simulink model "Pv"  (R2015a)
settings: Solver=ode45  StartTime=0.0  StopTime=3  RelTol=1e-3
values from neighbouring files (symbols this model uses):
  Iph_array = Iph*Npar    (= 29.801)    [sunpower305.m]
  Isat_array = Isat*Npar    (= 5.8765e-08)    [sunpower305.m]
  Rp_array = Rp*Nser/Npar    (= 198.702)    [sunpower305.m]
  Rs_array = Rs*Nser/Npar    (= 0.0075996)    [sunpower305.m]
  Ts = Ts_Power    (= 1e-06)    [sunpower305.m]
  Ts_Control = 100e-6    (= 0.0001)    [sunpower305.m]
  Ts_Power = 1e-6    (= 1e-06)    [sunpower305.m]
  VT_array = VT*Nser    (= 3.20466023218)    [sunpower305.m]
undefined symbols (not defined in the file or in its folder): sigbuilder_block
libraries: powerlib x16, simulink x2, powerlib_extras x1
settings Model: SimulationMode=accelerator  Creator=Limon  LastModifiedBy=Limon

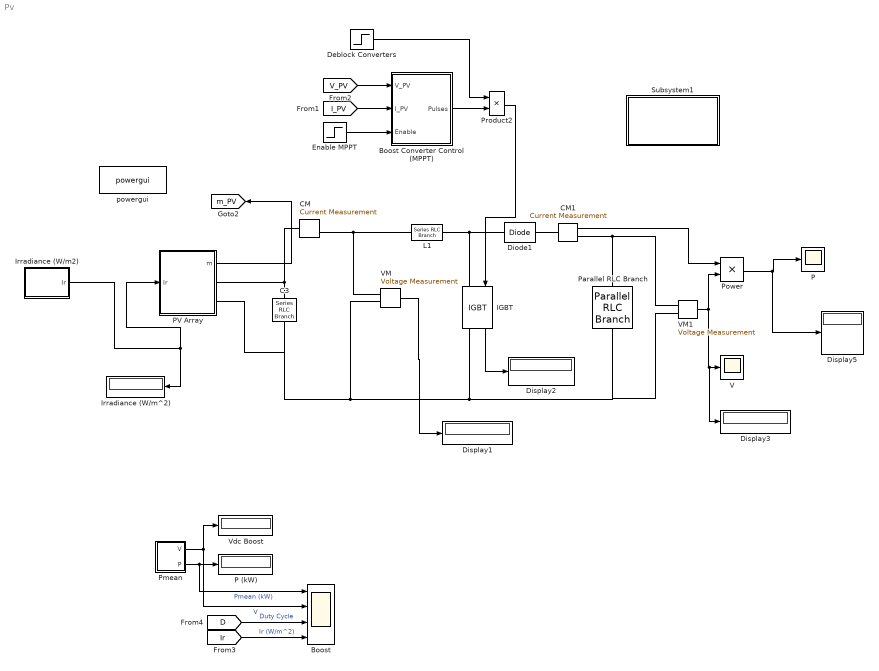
== system Pv ==
  Boost : Scope  NumInputPorts=4
      settings: TimeRange=3  YMin=0~-50~0~200  YMax=35~200~1~1000  SaveName=ScopeData_Boost  Decimation=100  SampleInput=on  SampleTime=Ts_Control
  Boost Converter Control (MPPT) : Subsystem
  C3 : powerlib/Elements/Series RLC Branch  LConnTagsString=__new0  RConnTagsString=__new0  BranchType=C  Resistance=1.0  Inductance=1.0  SetiL0=off  InitialCurrent=0  Capacitance=100e-6  Setx0=off  InitialVoltage=0  Measurements=Branch voltage
  CM : powerlib/Measurements/Current Measurement  PhasorSimulation=off  OutputType=Complex  PSBequivalent=0
  CM1 : powerlib/Measurements/Current Measurement  PhasorSimulation=off  OutputType=Complex  PSBequivalent=0
  Deblock Converters : Step  Time=0.05  SampleTime=0
  Diode1 : powerlib/Power Electronics/Diode  Ron=1e-4  Lon=0  Vf=0  IC=0  UseSnubber=off  Rs=inf  Cs=inf  Measurements=off
  Display{1..3,5} (4 alike) : Display
  Enable MPPT : Step  Time=0.4  SampleTime=0
  IGBT : powerlib/Power Electronics/IGBT  Ron=0.001  Lon=0  Vf=0  Tf=0  Tt=0  IC=0  Rs=1e5  Cs=inf  Measurements=on
  "Irradiance (W/m2) " : Subsystem  Tag=STV Subsys  LoadFcn=sigbuilder_block('load');  StartFcn=sigbuilder_block('start');  StopFcn=sigbuilder_block('stop');  ClipboardFcn=sigbuilder_block('clipboard');  mask(Sigbuilder block){}
      mask help: Sigbuilder GUI
      mask init:
      | if ~strcmp(get_param(bdroot(gcbh),'SimulationStatus'),'stopped') tuvar = sigbuilder_block('maskInit'); end
      settings: CopyFcn=sigbuilder_block('copy');  DeleteFcn=sigbuilder_block('delete');  ModelCloseFcn=sigbuilder_block('modelClose');  PreSaveFcn=sigbuilder_block('preSave');  PauseFcn=sigbuilder_block('pause')  ContinueFcn=sigbuilder_block('continue')  NameChangeFcn=sigbuilder_block('namechange');  OpenFcn=sigbuilder_block('open',[9 136.5 954 513.75 ]);  CloseFcn=sigbuilder_block('close');
      mask Display: plot(0,0,100,100,[10,10,40,40,10],[80,20,20,80,80],[40,10],[50,50], [40,27,10],[65,72,56],[40,25,25,10],[28,28,43,43]);
  Irradiance (W/m^2) : Display
      settings: Format=bank  Decimation=1000
  L1 : powerlib/Elements/Series RLC Branch  LConnTagsString=__new0  RConnTagsString=__new0  BranchType=RL  Resistance=0.005  Inductance=5e-3  SetiL0=off  InitialCurrent=0  Capacitance=1e-6  Setx0=off  InitialVoltage=0  Measurements=None
  P : Scope
      settings: TimeRange=1  YMin=-0  YMax=6e+06  SaveName=ScopeData4
  "P (kW) " : Display
      settings: Format=bank  Decimation=2000
  PV Array : Subsystem
  Parallel RLC Branch : powerlib/Elements/Parallel RLC Branch  LConnTagsString=a  RConnTagsString=__new0  BranchType=RC  Resistance=1e3  Inductance=1e-3  SetiL0=off  InitialCurrent=0  Capacitance=1e-6  Setx0=off  InitialVoltage=0  Measurements=None
  Pmean : Subsystem
  Power : Product
  Product2 : Product  RndMeth=Zero
  Subsystem1 : Subsystem
      mask Display: disp('Measurements')
  V : Scope
      settings: TimeRange=1  YMin=0  YMax=2100  SaveName=ScopeData2
  VM : powerlib/Measurements/Voltage Measurement  PhasorSimulation=off  OutputType=Complex  PSBequivalent=0
  VM1 : powerlib/Measurements/Voltage Measurement  PhasorSimulation=off  OutputType=Complex  PSBequivalent=0
  Vdc Boost : Display
      settings: Format=bank  Decimation=2000
  powergui : powerlib/powergui  Priority=1  SimulationMode=Discrete  SolverType=Tustin  SampleTime=Ts_Power  frequency=60  SPID=off  DisableSnubberDevices=off  DisableRonSwitches=off  DisableVfSwitches=off  SwTol=0  DisplayEquations=off  Interpol=off  methode=off  Ts=0  FunctionMessages=off  echomessages=off  HookPort=off  EnableUseOfTLC=off  x0status=blocks  frequencyindice=0  Pbase=100e6  ErrMax=1e-4  Iterations=50  UnitsV=kV  UnitsW=MW  buscounter=0  RestoreLinks=warning  ResistiveCurrentMeasurement=off  Frange=[0:2:500]  Ylog=off  Xlog=on  ShowGrid=off  save=off  variable=ZData  structure=0  ZoomFFT=on  StartTime=0.0  cycles=1  DisplayStyle=1  fundamental=60  FreqAxis=off  MaxFrequency=1000  frequencyindicesteady=1  RmsSteady=1  display=off
  tag scope: m_PV=global
  wires:
  IGBT/1 -> Display2/1
  VM1/1 -> Power/2, Display3/1, V/1
  CM1/1 -> Power/1
  Power/1 -> Display5/1, P/1
  VM/1 -> Display1/1
  "Irradiance (W/m2) "/1(Ir) -> Irradiance (W/m^2)/1, PV Array/1(Ir)
  PV Array/1(m) -> [m_PV]
  Pmean/2(P) -> "P (kW) "/1, Boost/1  "Pmean (kW)"
  Pmean/1(V) -> Vdc Boost/1, Boost/2  "V"
  [D] -> Boost/3  "Duty Cycle"
  [Ir] -> Boost/4  "Ir (W/m^2)"
  Product2/1 -> IGBT/1
  Deblock Converters/1 -> Product2/1
  Boost Converter Control (MPPT)/1(Pulses) -> Product2/2
  [V_PV] -> Boost Converter Control (MPPT)/1(V_PV)
  [I_PV] -> Boost Converter Control (MPPT)/2(I_PV)
  Enable MPPT/1 -> Boost Converter Control (MPPT)/3(Enable)
  connections:
  C3/LConn1 -- CM/LConn1 -- PV Array/RConn1
  VM/LConn2 -- PV Array/RConn2 -- C3/RConn1 -- VM1/LConn2 -- Parallel RLC Branch/RConn1 -- IGBT/RConn1
  IGBT/LConn1 -- L1/RConn1 -- Diode1/LConn1
  VM/LConn1 -- L1/LConn1 -- CM/RConn1
  CM1/LConn1 -- Diode1/RConn1
  Parallel RLC Branch/LConn1 -- VM1/LConn1 -- CM1/RConn1

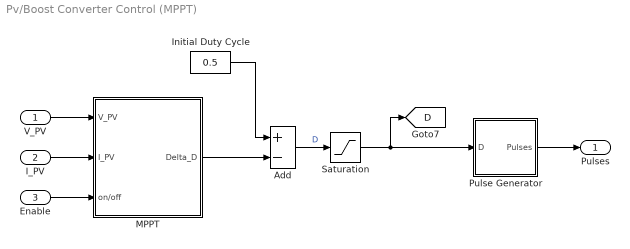
== system Pv/Boost Converter Control (MPPT) ==
  V_PV : Inport
  I_PV : Inport  Port=2
  Enable : Inport  Port=3
  Add : Sum  Inputs=+-
  Initial Duty Cycle : Constant  Value=0.5
  MPPT : Subsystem
  Pulse Generator : Subsystem  mask{Freq=5000}
      mask prompts: Freq "Frequency (Hz)"
  Saturation : Saturate  UpperLimit=1  LowerLimit=0
  Pulses : Outport
  tag scope: D=global
  wires:
  Initial Duty Cycle/1 -> Add/1
  MPPT/1(Delta_D) -> Add/2
  Add/1 -> Saturation/1  "D"
  Saturation/1 -> Pulse Generator/1(D), [D]
  Enable/1 -> MPPT/3(on/off)
  Pulse Generator/1(Pulses) -> Pulses/1
  I_PV/1 -> MPPT/2(I_PV)
  V_PV/1 -> MPPT/1(V_PV)

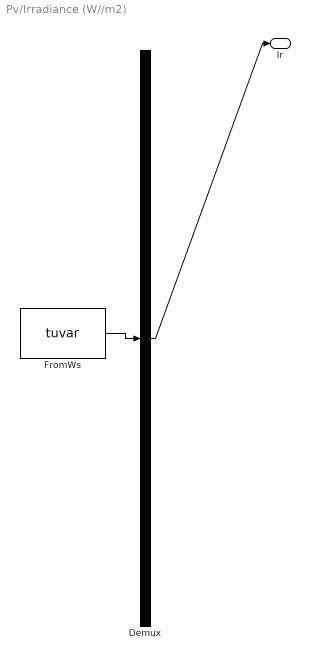
== system Pv/Irradiance (W//m2)  ==
  Demux : Demux  Tag=STV Demux  Outputs=1
  FromWs : FromWorkspace  Tag=STV FromWs  VariableName=tuvar  SampleTime=0
      SigBuilderData=|
      | common.afterFinalStr = 'Extrapolate'
      | common.sampleTime = '0'
      | dataSet(1).timeRange = [0 1]
      | dataSet(1).name = 'Constant Irradiance'
      | dataSet(2).timeRange = [0 1]
      | dataSet(2).name = 'Step Irradiance'
      | dataSet(3).timeRange = [0 3]
      | dataSet(3).name = 'Ramp-up/down Irradiance'
      | sbobj.Groups(1).Name = 'Constant Irradiance'
      | sbobj.Groups(1).Signals.Name = 'Ir'
      | sbobj.Groups(1).Signals.XData = [0 1]
      | sbobj.Groups(1).Signals.YData = [1000 1000]
      | sbobj.Groups(1).TimeRange = [0 1]
      | sbobj.Groups(2).Name = 'Step Irradiance'
      | sbobj.Groups(2).Signals.Name = 'Ir'
      | sbobj.Groups(2).Signals.XData = [0 0.501 0.51 0.69 0.7 1]
      | sbobj.Groups(2).Signals.YData = [1000 1000 250 250 1000 1000]
      | sbobj.Groups(2).TimeRange = [0 1]
      | sbobj.Groups(3).Name = 'Ramp-up/down Irradiance'
      | sbobj.Groups(3).Signals.Name = 'Ir'
      | sbobj.Groups(3).Signals.XData = [0 0.7 1.2 1.5 2 2.3 2.35 2.65 2.7 3]
      | sbobj.Groups(3).Signals.YData = [1000 1000 250 250 1000 1000 250 250 1000 1000]
      | sbobj.Groups(3).TimeRange = [0 3]
  Ir : Outport  Tag=STV Outport
  wires:
  Demux/1 -> Ir/1
  FromWs/1 -> Demux/1

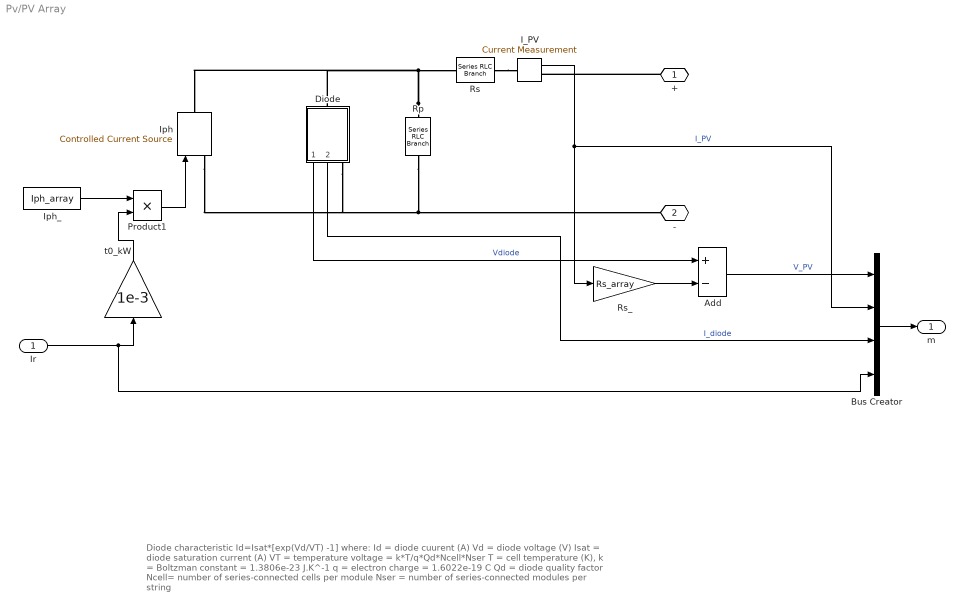
== system Pv/PV Array ==
  note: Diode characteristic
      | Id=Isat*[exp(Vd/VT) -1]
      |
      | where:
      | Id = diode cuurent (A)
      | Vd = diode voltage (V)
      | Isat = diode saturation current (A)
      | VT = temperature voltage = k*T/q*Qd*Ncell*Nser
      |
      | T = cell temperature (K),
      | k = Boltzman constant = 1.3806e-23 J.K^-1
      | q = electron charge = 1.6022e-19 C
      | Qd = diode quality factor
      | Ncell= number of series-connected cells per module
      | Nser = number of series-connected modules per string
  Ir : Inport
  Add : Sum  Inputs=+-
  Bus Creator : BusCreator
  Diode : Subsystem
      mask Display:
      | plot(-75,-50,100,150, [-15 -15 43 -15 -15 -75],[50 8 50 92 50 50], ...
      |     [43 43],[8 94],[100 43], [50 50])
  I_PV : powerlib/Measurements/Current Measurement  PhasorSimulation=off  OutputType=Complex  PSBequivalent=0
  Iph : powerlib/Electrical Sources/Controlled Current Source  Initialize=on  Source_Type=AC  Amplitude=0  Phase=0  Frequency=0  Measurements=None
  Iph_ : Constant  Value=Iph_array
  Product1 : Product  Inputs=**  RndMeth=Zero
  Rp : powerlib/Elements/Series RLC Branch  LConnTagsString=__new0  RConnTagsString=__new0  BranchType=R  Resistance=Rp_array  Inductance=1e-3  SetiL0=off  InitialCurrent=0  Capacitance=1e-6  Setx0=off  InitialVoltage=0  Measurements=Branch current
  Rs : powerlib/Elements/Series RLC Branch  LConnTagsString=__new0  RConnTagsString=__new0  BranchType=R  Resistance=Rs_array  Inductance=1e-3  SetiL0=off  InitialCurrent=0  Capacitance=1e-6  Setx0=off  InitialVoltage=0  Measurements=None
  Rs_ : Gain  Gain=Rs_array
  t0_kW : Gain  Gain=1e-3
  + : PMIOPort  Port=1  Side=Right
  - : PMIOPort  Port=2  Side=Right
  m : Outport
  wires:
  I_PV/1 -> Bus Creator/2, Rs_/1  "I_PV"
  Bus Creator/1 -> m/1
  Rs_/1 -> Add/2
  Diode/1(Vdiode) -> Add/1  "Vdiode"
  Diode/2(Idiode) -> Bus Creator/3  "I_diode"
  Add/1 -> Bus Creator/1  "V_PV"
  t0_kW/1 -> Product1/2
  Product1/1 -> Iph/1
  Iph_/1 -> Product1/1
  Ir/1 -> Bus Creator/4, t0_kW/1
  connections:
  +/RConn1 -- I_PV/RConn1
  Rs/LConn1 -- I_PV/LConn1
  Rp/LConn1 -- Rs/RConn1 -- Iph/RConn1 -- Diode/LConn1
  Rp/RConn1 -- Diode/RConn1 -- Iph/LConn1 -- -/RConn1

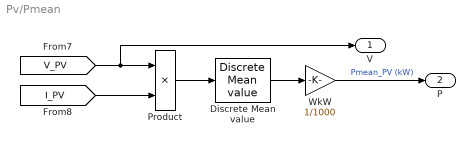
== system Pv/Pmean ==
  Discrete Mean value : powerlib_extras/Discrete Measurements/Discrete  Mean value  Freq=60  Vinit=0  Ts=Ts_Control
  Product : Product  RndMeth=Zero
  WkW : Gain  Gain=1/1000
  V : Outport
  P : Outport  Port=2
  wires:
  [V_PV] -> Product/1, V/1
  Product/1 -> Discrete Mean value/1
  [I_PV] -> Product/2
  WkW/1 -> P/1  "Pmean_PV (kW)"
  Discrete Mean value/1 -> WkW/1

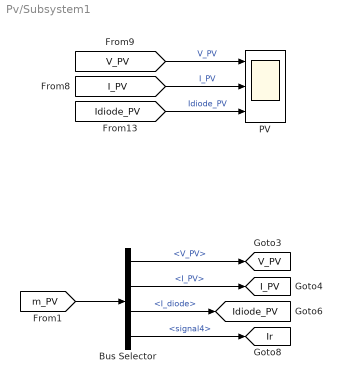
== system Pv/Subsystem1 ==
  Bus Selector : BusSelector  OutputSignals=V_PV,I_PV,I_diode,signal4
  PV : Scope  NumInputPorts=3
      settings: TimeRange=2  YMin=240~0~0  YMax=280~400~50  SaveName=ScopeData2  Decimation=100
  tag scope: I_PV=global, Idiode_PV=global, Ir=global, V_PV=global
  wires:
  [V_PV] -> PV/1  "V_PV"
  [I_PV] -> PV/2  "I_PV"
  [Idiode_PV] -> PV/3  "Idiode_PV"
  [m_PV] -> Bus Selector/1
  Bus Selector/1 -> [V_PV]  "<V_PV>"
  Bus Selector/2 -> [I_PV]  "<I_PV>"
  Bus Selector/3 -> [Idiode_PV]  "<I_diode>"
  Bus Selector/4 -> [Ir]  "<signal4>"

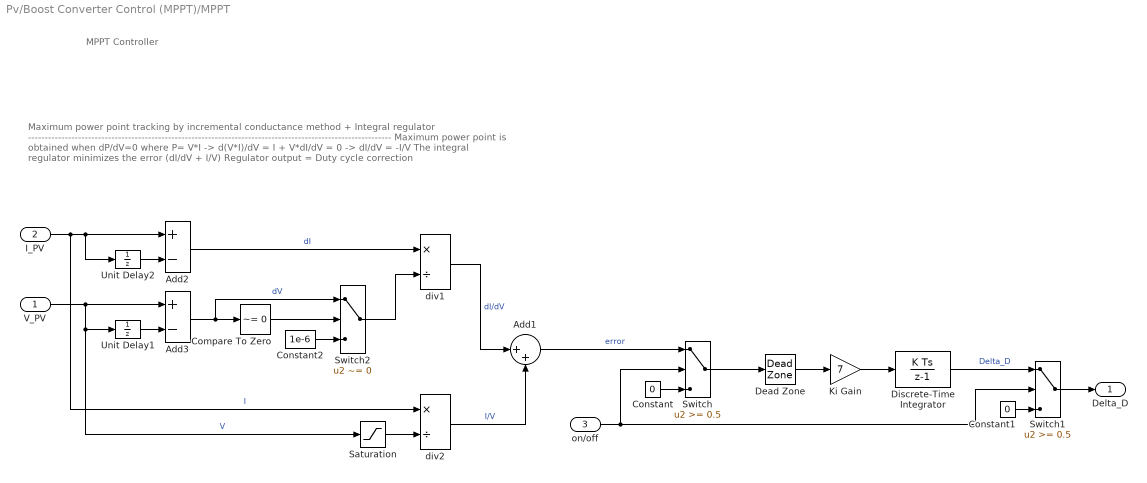
== system Pv/Boost Converter Control (MPPT)/MPPT ==
  note: Maximum power point tracking by incremental conductance method + Integral regulator
      | -------------------------------------------------------------------------------------------------------------
      | Maximum power point is obtained when dP/dV=0  where P= V*I
      | -> d(V*I)/dV = I + V*dI/dV = 0
      | -> dI/dV = -I/V
      | The integral regulator minimizes the error (dI/dV + I/V)
      | Regulator output = Duty cycle correction
  note: MPPT Controller
  V_PV : Inport
  I_PV : Inport  Port=2
  on/off : Inport  Port=3
  Add1 : Sum  Inputs=|++
  Add2 : Sum  Inputs=+-
  Add3 : Sum  Inputs=+-
  Compare To Zero : simulink/Logic and Bit Operations/Compare To Zero  relop=~=  OutDataTypeStr=uint8
  Constant : Constant  Value=0
  Constant1 : Constant  Value=0
  Constant2 : Constant  Value=1e-6
  Dead Zone : DeadZone  LowerValue=-0.02  UpperValue=+0.02  SaturateOnIntegerOverflow=on
  Discrete-Time Integrator : DiscreteIntegrator  gainval=1  SampleTime=Ts_Control  LimitOutput=on  UpperSaturationLimit=1  LowerSaturationLimit=-1
  Ki Gain : Gain  Gain=7
  Saturation : Saturate  UpperLimit=inf  LowerLimit=eps
  Switch : Switch  Threshold=0.5
  Switch1 : Switch  Threshold=0.5
  Switch2 : Switch  Criteria=u2 ~= 0
  Unit Delay1 : UnitDelay  SampleTime=Ts_Control
  Unit Delay2 : UnitDelay  SampleTime=Ts_Control
  div1 : Product  Inputs=*/  RndMeth=Zero
  div2 : Product  Inputs=*/  RndMeth=Zero
  Delta_D : Outport
  wires:
  V_PV/1 -> Add3/1, Saturation/1, Unit Delay1/1  "V"
  div1/1 -> Add1/1  "dI/dV"
  Constant/1 -> Switch/3
  Switch/1 -> Dead Zone/1
  Unit Delay1/1 -> Add3/2
  Compare To Zero/1 -> Switch2/2
  Switch2/1 -> div1/2
  Constant2/1 -> Switch2/3
  I_PV/1 -> Unit Delay2/1, Add2/1, div2/1  "I"
  Unit Delay2/1 -> Add2/2
  Add3/1 -> Compare To Zero/1, Switch2/1  "dV"
  Add2/1 -> div1/1  "dI"
  Saturation/1 -> div2/2
  div2/1 -> Add1/2  "I/V"
  Add1/1 -> Switch/1  "error"
  Dead Zone/1 -> Ki Gain/1
  Constant1/1 -> Switch1/3
  Discrete-Time Integrator/1 -> Switch1/1  "Delta_D"
  Switch1/1 -> Delta_D/1
  on/off/1 -> Switch/2, Switch1/2
  Ki Gain/1 -> Discrete-Time Integrator/1

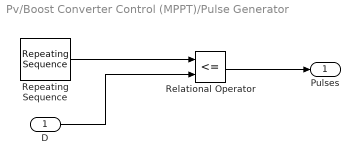
== system Pv/Boost Converter Control (MPPT)/Pulse Generator ==
  D : Inport
  Relational Operator : RelationalOperator  Operator=<=  OutDataTypeStr=boolean
  Repeating Sequence : simulink/Sources/Repeating Sequence  rep_seq_t="[0  1/Freq]"  rep_seq_y=[0 1]
  Pulses : Outport
  wires:
  D/1 -> Relational Operator/2
  Relational Operator/1 -> Pulses/1
  Repeating Sequence/1 -> Relational Operator/1

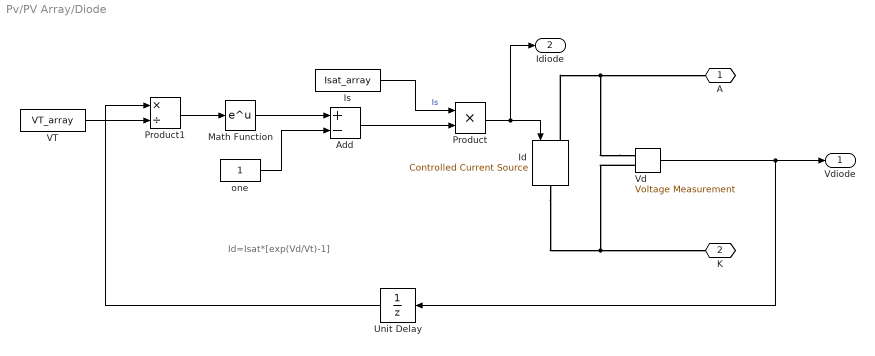
== system Pv/PV Array/Diode ==
  note: Id=Isat*[exp(Vd/Vt)-1]
  Add : Sum  Inputs=+-
  Id : powerlib/Electrical Sources/Controlled Current Source  Initialize=on  Source_Type=AC  Amplitude=0  Phase=0  Frequency=0  Measurements=None
  Is : Constant  Value=Isat_array
  Math Function : Math  SaturateOnIntegerOverflow=on
  Product : Product  RndMeth=Zero
  Product1 : Product  Inputs=*/  RndMeth=Zero
  Unit Delay : UnitDelay  SampleTime=Ts
  VT : Constant  Value=VT_array
  Vd : powerlib/Measurements/Voltage Measurement  PhasorSimulation=off  OutputType=Complex  PSBequivalent=0
  one : Constant
  A : PMIOPort  Port=1  Side=Left
  K : PMIOPort  Port=2  Side=Right
  Vdiode : Outport
  Idiode : Outport  Port=2
  wires:
  Product/1 -> Idiode/1, Id/1
  Vd/1 -> Vdiode/1, Unit Delay/1
  Is/1 -> Product/1  "Is"
  Product1/1 -> Math Function/1
  one/1 -> Add/2
  Add/1 -> Product/2
  VT/1 -> Product1/2
  Unit Delay/1 -> Product1/1
  Math Function/1 -> Add/1
  connections:
  Id/RConn1 -- K/RConn1 -- Vd/LConn2
  Vd/LConn1 -- A/RConn1 -- Id/LConn1
